simulink model "Lab1_419_sim5"  (R2023b)
settings: Solver=VariableStepAuto  StartTime=0.0  StopTime=10.0  RelTol=1e-9
settings Model: Creator=julia  LastModifiedBy=julia

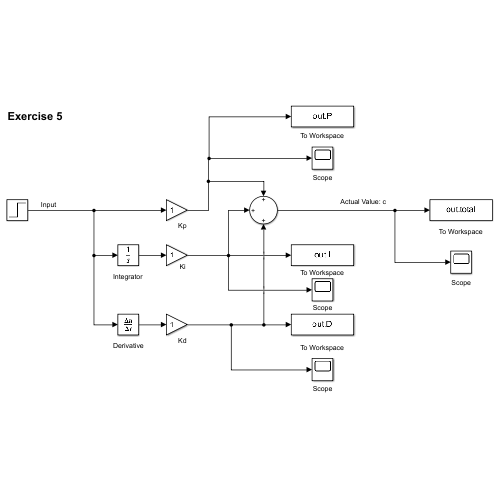
[thumbnail: Simulink's stored preview of the top-level diagram]
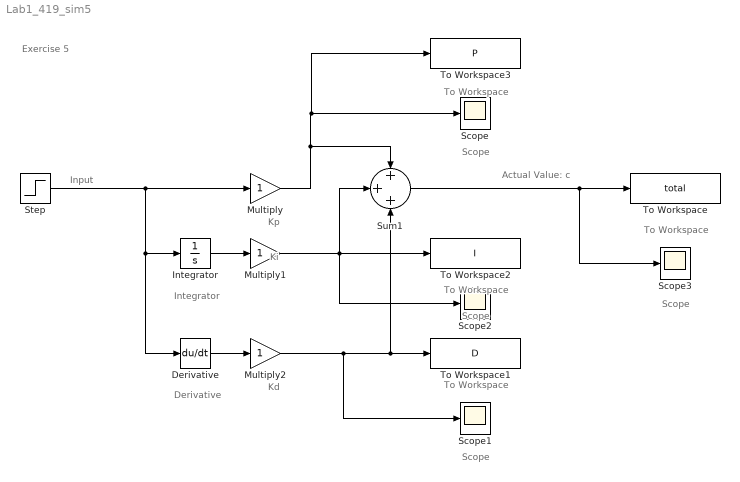
== system Lab1_419_sim5 ==
  note: Scope
  note: Exercise 5
  note: To Workspace
  note: Kp
  note: Ki
  note: Kd
  note: Actual Value: c
  note: Derivative
  note: Integrator
  note: Input
  note: To Workspace
  note: To Workspace
  note: To Workspace
  note: Scope
  note: Scope
  note: Scope
  Derivative : Derivative  CoefficientInTFapproximation=0
  Integrator : Integrator
  Multiply : Gain
  Multiply1 : Gain
  Multiply2 : Gain
  Scope{,1..3} (4 alike) : Scope
  Step : Step  SampleTime=0.001
  Sum1 : Sum  Inputs=+++
  To Workspace : ToWorkspace  VariableName=total  SampleTime=-1
  To Workspace1 : ToWorkspace  VariableName=D  SampleTime=-1
  To Workspace2 : ToWorkspace  VariableName=I  SampleTime=-1
  To Workspace3 : ToWorkspace  VariableName=P  SampleTime=-1
  wires:
  Step/1 -> Derivative/1, Integrator/1, Multiply/1
  Integrator/1 -> Multiply1/1
  Derivative/1 -> Multiply2/1
  Multiply/1 -> To Workspace3/1, Scope/1, Sum1/1
  Multiply1/1 -> Scope2/1, To Workspace2/1, Sum1/2
  Sum1/1 -> Scope3/1, To Workspace/1
  Multiply2/1 -> Scope1/1, To Workspace1/1, Sum1/3
